simulink model "question10_2018"  (R2018b)
settings: Solver=VariableStepAuto  StartTime=0.0  StopTime=10.0  RelTol=1e-3
values from neighbouring files (symbols this model uses):
  A = [ 0 1 0 0 ... (first row only)    [Alt_Industrial_plant.m]    (also in IndustrialPlant.m; ObserverExample.m = [0 1 0; 980  0  -2.8; 0 0 -100]; OldProject.m = [0 1 0 0 ;-491 0 -282.45 0; 0 0 0 1;1488 0 885.65 0]; observerWorkingExample.m = [0, 0, 1, 0)
  Ad = sys_d.a    [Alt_Industrial_plant.m]    (also in observerWorkingExample.m)
  B = [0; 1/Jd; 0; 0]    [Alt_Industrial_plant.m]    (also in IndustrialPlant.m; ObserverExample.m = [ 0; 0; 100]; OldProject.m = [0;82.33;0;-235.29]; observerWorkingExample.m = [0; 0; 1/mc; 1/(L*mc)])
  Bd = sys_d.b    [Alt_Industrial_plant.m]    (also in observerWorkingExample.m)
  Cd = sys_d.c    [Alt_Industrial_plant.m]    (also in observerWorkingExample.m)
  K = acker(A,B,des_poles)    [Alt_Industrial_plant.m]    (also in ObserverExample.m = place(A,B,[p1 p2 p3]); OldProject.m = place(A,B,Pole_fb); observerWorkingExample.m)
  K_d = acker(Ad,Bd,des_poles_d)    [Alt_Industrial_plant.m]    (also in observerWorkingExample.m)
  K_lqr = lqr(A,B,Q,R)    [observerWorkingExample.m]
  Ob = place(A',C,obs_poles)    [Alt_Industrial_plant.m]    (also in observerWorkingExample.m = acker(Ad',Cd',des_poles_d))
  Ts = 0.1    [Alt_Industrial_plant.m]    (also in observerWorkingExample.m)
  x0 = [0;15*pi/180;0;0]    [Alt_Industrial_plant.m]    (also in ObserverExample.m = [0.01 0.5 -5]; observerWorkingExample.m = [0;5*pi/180;0;0])
settings Model: Creator=Yaipiti  LastModifiedBy=Yaipiti
settings DataIOCC: ReturnWorkspaceOutputs=on

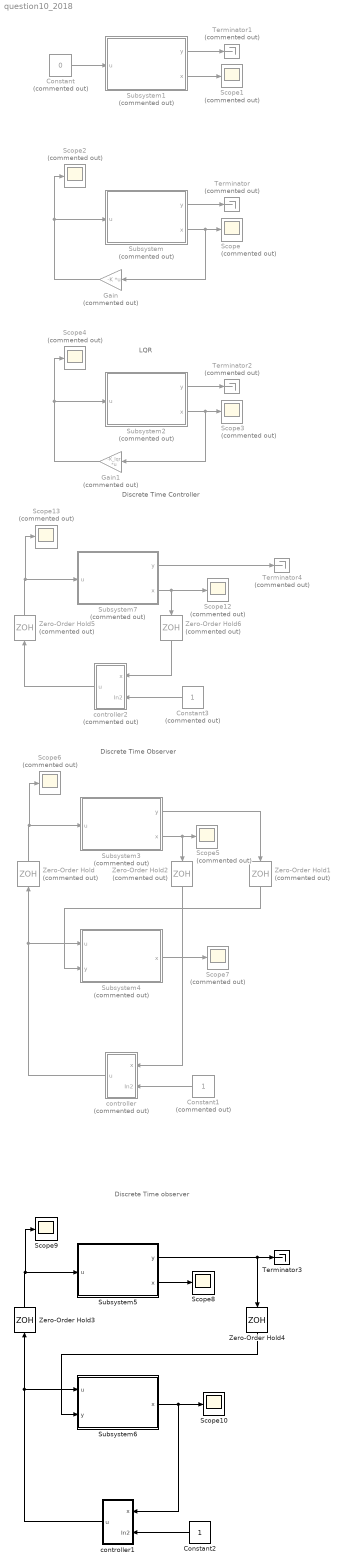
== system question10_2018 ==
  note: LQR
  note: Discrete Time Controller
  note: Discrete Time observer
  note: Discrete Time Observer
  Constant : Constant  Commented=on  Value=0
  Constant1 : Constant  Commented=on
  Constant2 : Constant
  Constant3 : Constant  Commented=on
  Gain : Gain  Commented=on  Gain=-K  Multiplication=Matrix(K*u)
  Gain1 : Gain  Commented=on  Gain=-K_lqr  Multiplication=Matrix(K*u)
  Scope{,1..7,12..13} (10 alike) : Scope  Commented=on
  Scope10 : Scope
  Scope8 : Scope
  Scope9 : Scope
  Subsystem : Subsystem  Commented=on
  Subsystem1 : Subsystem  Commented=on
  Subsystem2 : Subsystem  Commented=on
  Subsystem3 : Subsystem  Commented=on
  Subsystem4 : Subsystem  Commented=on
  Subsystem5 : Subsystem
  Subsystem6 : Subsystem
  Subsystem7 : Subsystem  Commented=on
  Terminator{,1..2,4} (4 alike) : Terminator  Commented=on
  Terminator3 : Terminator
  Zero-Order Hold{,1..2,5..6} (5 alike) : ZeroOrderHold  Commented=on  SampleTime=Ts
  Zero-Order Hold3 : ZeroOrderHold  SampleTime=Ts
  Zero-Order Hold4 : ZeroOrderHold  SampleTime=Ts
  controller : Subsystem  Commented=on
  controller1 : Subsystem
  controller2 : Subsystem  Commented=on
  wires:
  Subsystem/2(x) -> Gain/1, Scope/1
  Subsystem/1(y) -> Terminator/1
  Gain/1 -> Scope2/1, Subsystem/1(u)
  Subsystem1/1(y) -> Terminator1/1
  Subsystem1/2(x) -> Scope1/1
  Constant/1 -> Subsystem1/1(u)
  Subsystem2/1(y) -> Terminator2/1
  Gain1/1 -> Scope4/1, Subsystem2/1(u)
  Subsystem2/2(x) -> Gain1/1, Scope3/1
  Subsystem3/1(y) -> Zero-Order Hold1/1
  Subsystem3/2(x) -> Zero-Order Hold2/1, Scope5/1
  controller/1(u) -> Subsystem4/1(u), Zero-Order Hold/1
  Constant1/1 -> controller/2(In2)
  Zero-Order Hold/1 -> Scope6/1, Subsystem3/1(u)
  Zero-Order Hold1/1 -> Subsystem4/2(y)
  Zero-Order Hold2/1 -> controller/1(x)
  Subsystem4/1(x) -> Scope7/1
  Subsystem6/1(x) -> controller1/1(x), Scope10/1
  Zero-Order Hold4/1 -> Subsystem6/2(y)
  Subsystem5/1(y) -> Terminator3/1, Zero-Order Hold4/1
  Zero-Order Hold3/1 -> Scope9/1, Subsystem5/1(u)
  Subsystem5/2(x) -> Scope8/1
  Constant2/1 -> controller1/2(In2)
  controller1/1(u) -> Subsystem6/1(u), Zero-Order Hold3/1
  Zero-Order Hold5/1 -> Scope13/1, Subsystem7/1(u)
  Constant3/1 -> controller2/2(In2)
  controller2/1(u) -> Zero-Order Hold5/1
  Zero-Order Hold6/1 -> controller2/1(x)
  Subsystem7/1(y) -> Terminator4/1
  Subsystem7/2(x) -> Scope12/1, Zero-Order Hold6/1

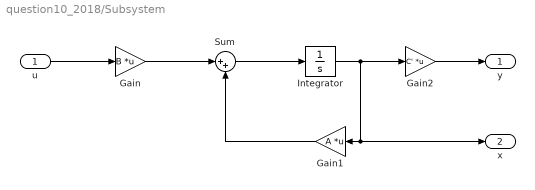
== system question10_2018/Subsystem ==
  u : Inport
  Gain : Gain  Gain=B  Multiplication=Matrix(K*u)
  Gain1 : Gain  Gain=A  Multiplication=Matrix(K*u)
  Gain2 : Gain  Gain=C'  Multiplication=Matrix(K*u)
  Integrator : Integrator  InitialCondition=x0
  Sum : Sum  Inputs=|++
  y : Outport
  x : Outport  Port=2
  wires:
  Gain/1 -> Sum/1
  Sum/1 -> Integrator/1
  Gain1/1 -> Sum/2
  u/1 -> Gain/1
  Gain2/1 -> y/1
  Integrator/1 -> Gain2/1, x/1, Gain1/1

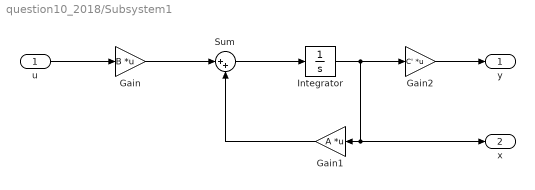
== system question10_2018/Subsystem1 ==
  u : Inport
  Gain : Gain  Gain=B  Multiplication=Matrix(K*u)
  Gain1 : Gain  Gain=A  Multiplication=Matrix(K*u)
  Gain2 : Gain  Gain=C'  Multiplication=Matrix(K*u)
  Integrator : Integrator  InitialCondition=x0
  Sum : Sum  Inputs=|++
  y : Outport
  x : Outport  Port=2
  wires:
  Gain/1 -> Sum/1
  Sum/1 -> Integrator/1
  Gain1/1 -> Sum/2
  u/1 -> Gain/1
  Gain2/1 -> y/1
  Integrator/1 -> Gain2/1, x/1, Gain1/1

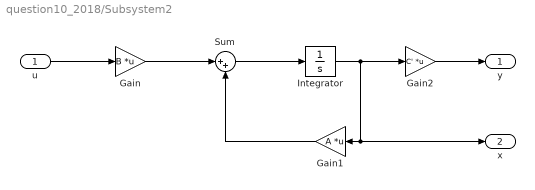
== system question10_2018/Subsystem2 ==
  u : Inport
  Gain : Gain  Gain=B  Multiplication=Matrix(K*u)
  Gain1 : Gain  Gain=A  Multiplication=Matrix(K*u)
  Gain2 : Gain  Gain=C'  Multiplication=Matrix(K*u)
  Integrator : Integrator  InitialCondition=x0
  Sum : Sum  Inputs=|++
  y : Outport
  x : Outport  Port=2
  wires:
  Gain/1 -> Sum/1
  Sum/1 -> Integrator/1
  Gain1/1 -> Sum/2
  u/1 -> Gain/1
  Gain2/1 -> y/1
  Integrator/1 -> Gain2/1, x/1, Gain1/1

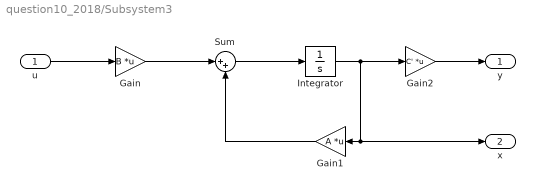
== system question10_2018/Subsystem3 ==
  u : Inport
  Gain : Gain  Gain=B  Multiplication=Matrix(K*u)
  Gain1 : Gain  Gain=A  Multiplication=Matrix(K*u)
  Gain2 : Gain  Gain=C'  Multiplication=Matrix(K*u)
  Integrator : Integrator  InitialCondition=x0
  Sum : Sum  Inputs=|++
  y : Outport
  x : Outport  Port=2
  wires:
  Gain/1 -> Sum/1
  Sum/1 -> Integrator/1
  Gain1/1 -> Sum/2
  u/1 -> Gain/1
  Gain2/1 -> y/1
  Integrator/1 -> Gain2/1, x/1, Gain1/1

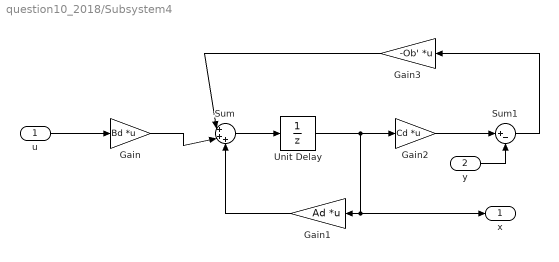
== system question10_2018/Subsystem4 ==
  u : Inport
  y : Inport  Port=2
  Gain : Gain  Gain=Bd  Multiplication=Matrix(K*u)
  Gain1 : Gain  Gain=Ad  Multiplication=Matrix(K*u)
  Gain2 : Gain  Gain=Cd  Multiplication=Matrix(K*u)
  Gain3 : Gain  Gain=-Ob'  Multiplication=Matrix(K*u)
  Sum : Sum  Inputs=|+++
  Sum1 : Sum  Inputs=|+-
  Unit Delay : UnitDelay  InitialCondition=x0*0  SampleTime=-1  HasFrameUpgradeWarning=on
  x : Outport
  wires:
  u/1 -> Gain/1
  Unit Delay/1 -> Gain2/1, x/1, Gain1/1
  Sum/1 -> Unit Delay/1
  y/1 -> Sum1/2
  Gain2/1 -> Sum1/1
  Sum1/1 -> Gain3/1
  Gain1/1 -> Sum/3
  Gain/1 -> Sum/2
  Gain3/1 -> Sum/1

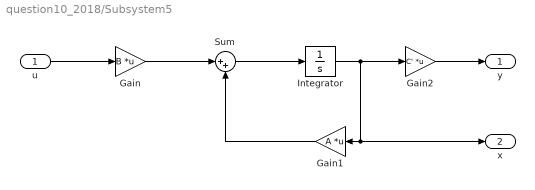
== system question10_2018/Subsystem5 ==
  u : Inport
  Gain : Gain  Gain=B  Multiplication=Matrix(K*u)
  Gain1 : Gain  Gain=A  Multiplication=Matrix(K*u)
  Gain2 : Gain  Gain=C'  Multiplication=Matrix(K*u)
  Integrator : Integrator  InitialCondition=x0
  Sum : Sum  Inputs=|++
  y : Outport
  x : Outport  Port=2
  wires:
  Gain/1 -> Sum/1
  Sum/1 -> Integrator/1
  Gain1/1 -> Sum/2
  u/1 -> Gain/1
  Gain2/1 -> y/1
  Integrator/1 -> Gain2/1, x/1, Gain1/1

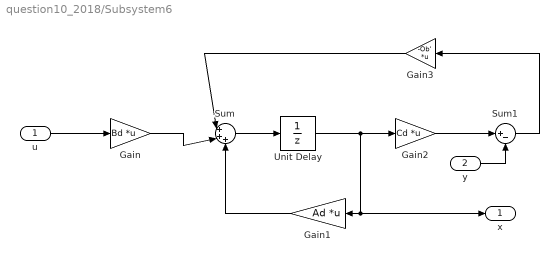
== system question10_2018/Subsystem6 ==
  u : Inport
  y : Inport  Port=2
  Gain : Gain  Gain=Bd  Multiplication=Matrix(K*u)
  Gain1 : Gain  Gain=Ad  Multiplication=Matrix(K*u)
  Gain2 : Gain  Gain=Cd  Multiplication=Matrix(K*u)
  Gain3 : Gain  Gain=-Ob'  Multiplication=Matrix(K*u)
  Sum : Sum  Inputs=|+++
  Sum1 : Sum  Inputs=|+-
  Unit Delay : UnitDelay  InitialCondition=x0*0  SampleTime=-1  HasFrameUpgradeWarning=on
  x : Outport
  wires:
  u/1 -> Gain/1
  Unit Delay/1 -> Gain2/1, x/1, Gain1/1
  Sum/1 -> Unit Delay/1
  y/1 -> Sum1/2
  Gain2/1 -> Sum1/1
  Sum1/1 -> Gain3/1
  Gain1/1 -> Sum/3
  Gain/1 -> Sum/2
  Gain3/1 -> Sum/1

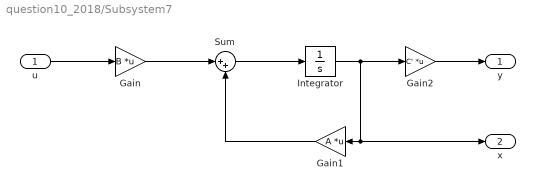
== system question10_2018/Subsystem7 ==
  u : Inport
  Gain : Gain  Gain=B  Multiplication=Matrix(K*u)
  Gain1 : Gain  Gain=A  Multiplication=Matrix(K*u)
  Gain2 : Gain  Gain=C'  Multiplication=Matrix(K*u)
  Integrator : Integrator  InitialCondition=x0
  Sum : Sum  Inputs=|++
  y : Outport
  x : Outport  Port=2
  wires:
  Gain/1 -> Sum/1
  Sum/1 -> Integrator/1
  Gain1/1 -> Sum/2
  u/1 -> Gain/1
  Gain2/1 -> y/1
  Integrator/1 -> Gain2/1, x/1, Gain1/1

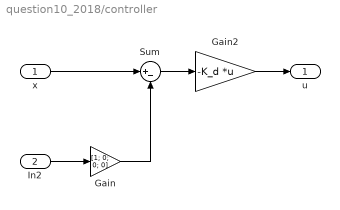
== system question10_2018/controller ==
  x : Inport
  In2 : Inport  Port=2
  Gain : Gain  Gain=[1; 0; 0; 0]
  Gain2 : Gain  Gain=-K_d  Multiplication=Matrix(K*u)
  Sum : Sum  Inputs=|+-
  u : Outport
  wires:
  Gain2/1 -> u/1
  x/1 -> Sum/1
  Sum/1 -> Gain2/1
  Gain/1 -> Sum/2
  In2/1 -> Gain/1

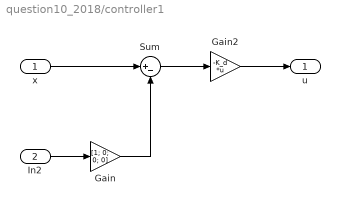
== system question10_2018/controller1 ==
  x : Inport
  In2 : Inport  Port=2
  Gain : Gain  Gain=[1; 0; 0; 0]
  Gain2 : Gain  Gain=-K_d  Multiplication=Matrix(K*u)
  Sum : Sum  Inputs=|+-
  u : Outport
  wires:
  Gain2/1 -> u/1
  x/1 -> Sum/1
  Sum/1 -> Gain2/1
  Gain/1 -> Sum/2
  In2/1 -> Gain/1

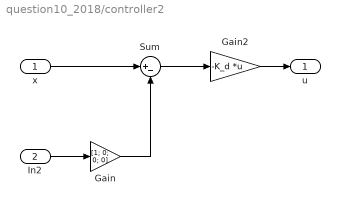
== system question10_2018/controller2 ==
  x : Inport
  In2 : Inport  Port=2
  Gain : Gain  Gain=[1; 0; 0; 0]
  Gain2 : Gain  Gain=-K_d  Multiplication=Matrix(K*u)
  Sum : Sum  Inputs=|+-
  u : Outport
  wires:
  Gain2/1 -> u/1
  x/1 -> Sum/1
  Sum/1 -> Gain2/1
  Gain/1 -> Sum/2
  In2/1 -> Gain/1
